simulink model "stateflow_scout"  (R2018a)
settings: Solver=VariableStepAuto  StartTime=0.0  StopTime=10.0  RelTol=1e-3
settings Model: Creator=Vahu  LastModifiedBy=Vahu

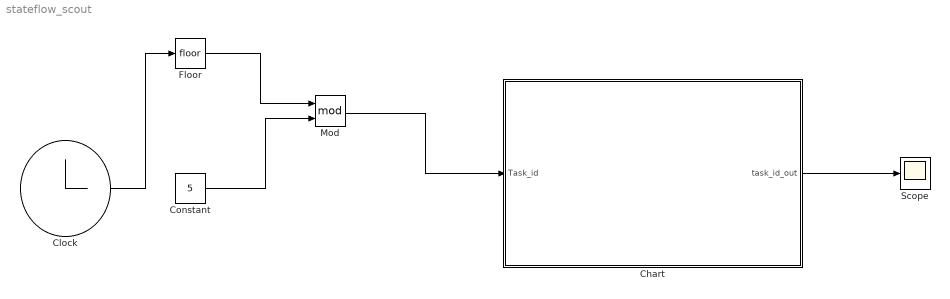
== system stateflow_scout ==
  Chart : Stateflow chart  TreatAsAtomicUnit=on
  Clock : Clock
  Constant : Constant  Value=5
  Floor : Rounding
  Mod : Math  Operator=mod  SaturateOnIntegerOverflow=on
  Scope : Scope
  wires:
  Clock/1 -> Floor/1
  Constant/1 -> Mod/2
  Floor/1 -> Mod/1
  Mod/1 -> Chart/1(Task_id)
  Chart/1(task_id_out) -> Scope/1

== stateflow chart stateflow_scout/Chart ==
  state sensor
    during: Task_id <= 3;
  state Referee
    entry: task_id_out = 1
    during: Task_id <= 2;
  state idle
    entry: task_id_out = 0
    during: Task_id <= 1
  state team_mate
    during: Task_id <= 4;
  state drive_decision
  (default) -> idle
  Referee -> sensor : [Task_id == 2]{task_id_out = 2}
  idle -> Referee : [Task_id == 1]{task_id_out = 1}
  sensor -> team_mate : [Task_id == 3]{task_id_out = 3}
  drive_decision -> idle : [Task_id == 0]{task_id_out = 0}
  team_mate -> drive_decision : [Task_id == 4]{task_id_out = 4}
  data: Task_id input; task_id_out output
